simulink model "Lab2init"  (R2022b)
settings: Solver=VariableStepAuto  StartTime=0.0  StopTime=50.0  RelTol=1e-3
values from neighbouring files (symbols this model uses):
  V = 100    [Laboratory2.m]
undefined symbols (not defined in the file or in its folder): c0, ci, Edr, k0, q
settings Model: Creator=fabian  LastModifiedBy=fabian

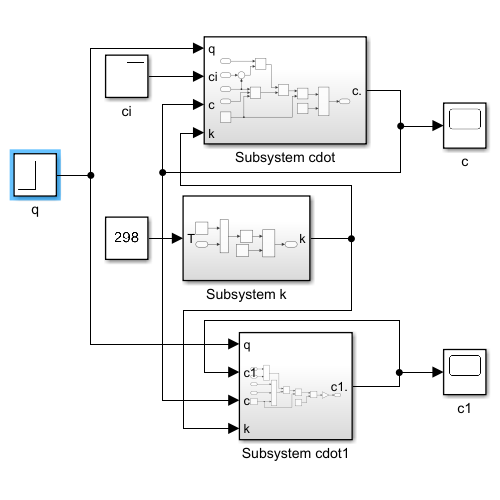
[thumbnail: Simulink's stored preview of the top-level diagram]
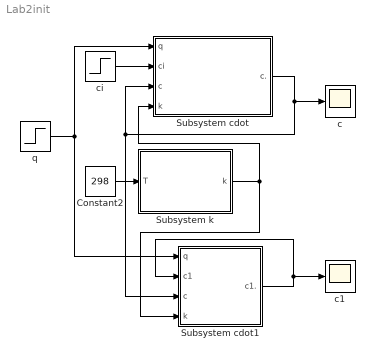
== system Lab2init ==
  Constant2 : Constant  Value=298
  Subsystem cdot : Subsystem
  Subsystem cdot1 : Subsystem
  Subsystem k : Subsystem
  c : Scope
  c1 : Scope
  ci : Step  Time=0  After=ci*1.1  SampleTime=0
  q : Step  Time=0  After=q  SampleTime=0
  wires:
  Subsystem cdot1/1(c1.) -> c1/1, Subsystem cdot1/2(c1)
  Subsystem cdot/1(c.) -> Subsystem cdot/3(c), Subsystem cdot1/3(c), c/1
  ci/1 -> Subsystem cdot/2(ci)
  Constant2/1 -> Subsystem k/1(T)
  Subsystem k/1(k) -> Subsystem cdot1/4(k), Subsystem cdot/4(k)
  q/1 -> Subsystem cdot1/1(q), Subsystem cdot/1(q)

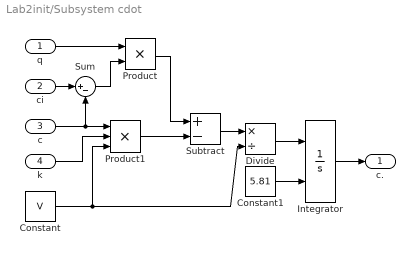
== system Lab2init/Subsystem cdot ==
  q : Inport
  ci : Inport  Port=2
  c : Inport  Port=3
  k : Inport  Port=4
  Constant : Constant  Value=V
  Constant1 : Constant  Value=5.81
  Divide : Product  Inputs=*/
  Integrator : Integrator  InitialConditionSource=external  InitialCondition=c0
  Product : Product
  Product1 : Product  Inputs=3
  Subtract : Sum  Inputs=+-
  Sum : Sum  Inputs=|+-
  c. : Outport
  wires:
  Product/1 -> Subtract/1
  Integrator/1 -> c./1
  Divide/1 -> Integrator/1
  Subtract/1 -> Divide/1
  q/1 -> Product/1
  Constant/1 -> Divide/2, Product1/3
  Sum/1 -> Product/2
  Constant1/1 -> Integrator/2
  c/1 -> Product1/1, Sum/2
  ci/1 -> Sum/1
  k/1 -> Product1/2
  Product1/1 -> Subtract/2

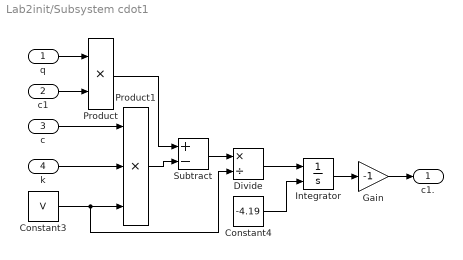
== system Lab2init/Subsystem cdot1 ==
  q : Inport
  c1 : Inport  Port=2
  c : Inport  Port=3
  k : Inport  Port=4
  Constant3 : Constant  Value=V
  Constant4 : Constant  Value=-4.19
  Divide : Product  Inputs=*/
  Gain : Gain  Gain=-1
  Integrator : Integrator  InitialConditionSource=external  InitialCondition=c0
  Product : Product
  Product1 : Product  Inputs=3
  Subtract : Sum  Inputs=+-
  c1. : Outport
  wires:
  Product/1 -> Subtract/1
  Constant3/1 -> Product1/3, Divide/2
  Product1/1 -> Subtract/2
  c/1 -> Product1/1
  Divide/1 -> Integrator/1
  Subtract/1 -> Divide/1
  q/1 -> Product/1
  k/1 -> Product1/2
  Constant4/1 -> Integrator/2
  c1/1 -> Product/2
  Gain/1 -> c1./1
  Integrator/1 -> Gain/1

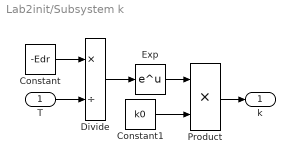
== system Lab2init/Subsystem k ==
  T : Inport
  Constant : Constant  Value=-Edr
  Constant1 : Constant  Value=k0
  Divide : Product  Inputs=*/
  Exp : Math
  Product : Product
  k : Outport
  wires:
  Exp/1 -> Product/1
  Constant/1 -> Divide/1
  Product/1 -> k/1
  Divide/1 -> Exp/1
  Constant1/1 -> Product/2
  T/1 -> Divide/2
